simulink model "quadrotor_nonlinear"  (R2026a)
settings: Solver=ode45  StopTime=4  MaxStep=0.01
model workspace (MAT data in the model file):
  x0 = [0; 0; -10; 0; 0; 0; 0; 0; 0; 0; 0; 0; 463.1; 463.1; 463.1; 463.1]
settings Model: Creator=ievge  LastModifiedBy=ievge

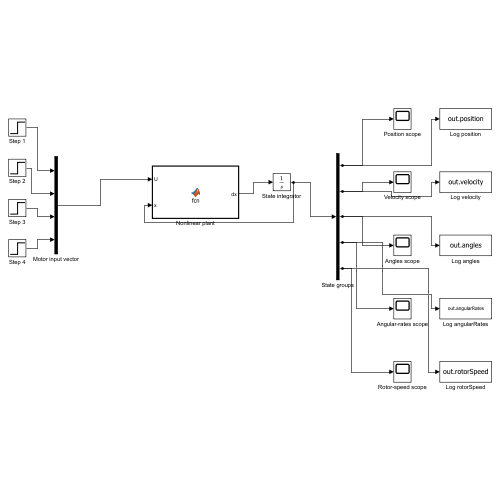
[thumbnail: Simulink's stored preview of the top-level diagram]
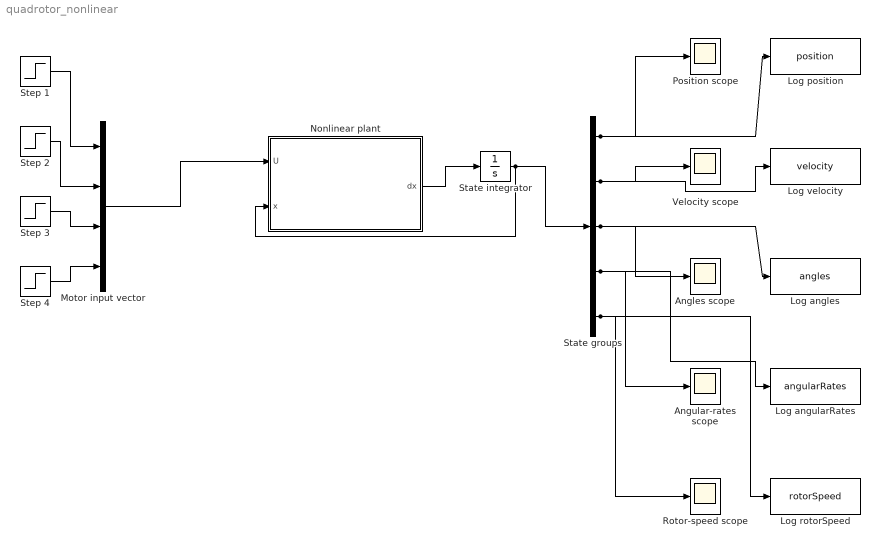
== system quadrotor_nonlinear ==
  Angles scope : Scope
  Angular-rates scope : Scope
  Log angles : ToWorkspace  VariableName=angles  SaveFormat=Timeseries  SampleTime=-1
  Log angularRates : ToWorkspace  VariableName=angularRates  SaveFormat=Timeseries  SampleTime=-1
  Log position : ToWorkspace  VariableName=position  SaveFormat=Timeseries  SampleTime=-1
  Log rotorSpeed : ToWorkspace  VariableName=rotorSpeed  SaveFormat=Timeseries  SampleTime=-1
  Log velocity : ToWorkspace  VariableName=velocity  SaveFormat=Timeseries  SampleTime=-1
  Motor input vector : Mux
  Nonlinear plant : MATLAB Function  TreatAsAtomicUnit=on
  Position scope : Scope
  Rotor-speed scope : Scope
  State groups : Demux  Outputs=[3 3 3 3 4]
  State integrator : Integrator  InitialCondition=x0
  Step {1..4} (4 alike) : Step  SampleTime=0
  Velocity scope : Scope
  wires:
  Step 1/1 -> Motor input vector/1
  Step 2/1 -> Motor input vector/2
  Step 3/1 -> Motor input vector/3
  Step 4/1 -> Motor input vector/4
  Motor input vector/1 -> Nonlinear plant/1(U)
  Nonlinear plant/1(dx) -> State integrator/1
  State integrator/1 -> Nonlinear plant/2(x), State groups/1
  State groups/1 -> Position scope/1, Log position/1
  State groups/2 -> Velocity scope/1, Log velocity/1
  State groups/3 -> Angles scope/1, Log angles/1
  State groups/4 -> Angular-rates scope/1, Log angularRates/1
  State groups/5 -> Rotor-speed scope/1, Log rotorSpeed/1

== matlab function quadrotor_nonlinear/Nonlinear plant ==
  data: U input size=[4 1]; dx output size=[16 1]; x input size=[16 1]
function dx = fcn(U, x)
%#codegen
g = 9.8100000000000005;
Ix = 0.0092999999999999992;
Iy = 0.0091999999999999998;
Iz = 0.015100000000000001;
Ip = 4.439e-05;
b = 1.5108e-05;
d = 4.4060000000000001e-07;
l = 0.23999999999999999;
m = 1.3211359852721711;
tau = 0.10000000000000001;
Kdc = 0.69999999999999996;
u_hover = 661.57142857142867;
Omega_min = 0;
Omega_max = 942.47779607693792;
u = x(4); v = x(5); w = x(6);
phi = x(7); th = x(8); ps = x(9);
p = x(10); q = x(11); r = x(12);
Om = x(13:16);
D = [cos(th)*cos(ps), cos(th)*sin(ps), -sin(th); sin(phi)*sin(th)*cos(ps)-cos(phi)*sin(ps), sin(phi)*sin(th)*sin(ps)+cos(phi)*cos(ps), sin(phi)*cos(th); cos(phi)*sin(th)*cos(ps)+sin(phi)*sin(ps), cos(phi)*sin(th)*sin(ps)-sin(phi)*cos(ps), cos(phi)*cos(th)];
pos_dot = D.' * [u; v; w];
Einv = [1, sin(phi)*tan(th), cos(phi)*tan(th); 0, cos(phi), -sin(phi); 0, sin(phi)/cos(th), cos(phi)/cos(th)];
ang_dot = Einv * [p; q; r];
T = b * sum(Om.^2);
Mx = l*b * (Om(2)^2 - Om(4)^2);
My = l*b * (Om(1)^2 - Om(3)^2);
Mz = d * (Om(2)^2 + Om(4)^2 - Om(1)^2 - Om(3)^2);
Hz = Ip * (Om(1) - Om(2) + Om(3) - Om(4));
u_dot = r*v - q*w - g*sin(th);
v_dot = p*w - r*u + g*cos(th)*sin(phi);
w_dot = q*u - p*v + g*cos(phi)*cos(th) - T/m;
p_dot = Mx/Ix - q*r*(Iz-Iy)/Ix - Hz*q/Ix;
q_dot = My/Iy - p*r*(Ix-Iz)/Iy + Hz*p/Iy;
r_dot = Mz/Iz;
omega_cmd = Kdc * (u_hover + U(:));
omega_cmd = min(max(omega_cmd, Omega_min), Omega_max);
Om_dot = (omega_cmd - Om) / tau;
dx = [pos_dot; u_dot; v_dot; w_dot; ang_dot; p_dot; q_dot; r_dot; Om_dot];
end
